simulink model "singlerobotlidarmap"  (R2021b)
settings: Solver=VariableStepAuto  StartTime=0.0  StopTime=10.0  RelTol=1e-3
InitFcn:
  | addpath("..");
  | initenv
libraries: mobileRoboticsLib x5, robotmobilelib x2
settings Model: Creator=yekin  LastModifiedBy=yekin

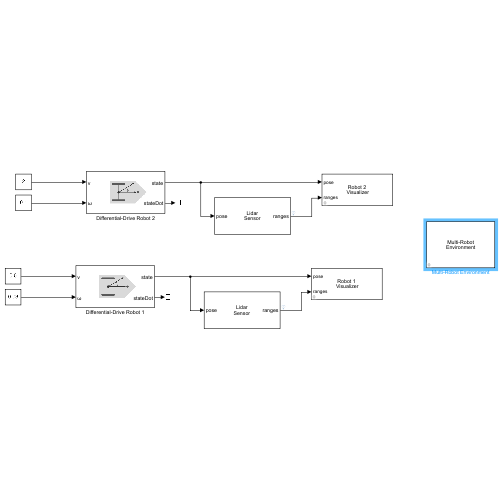
[thumbnail: Simulink's stored preview of the top-level diagram]
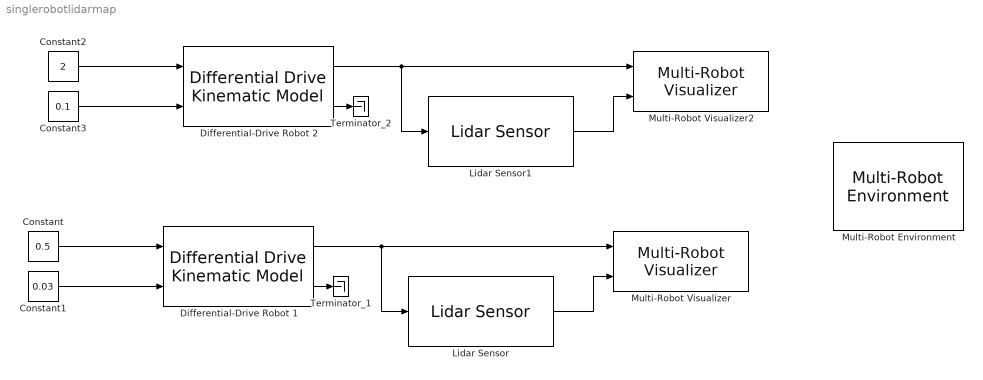
== system singlerobotlidarmap ==
  Constant : Constant  Value=0.5
  Constant1 : Constant  Value=0.03
  Constant2 : Constant  Value=2
  Constant3 : Constant  Value=0.1
  Differential-Drive Robot 1 : robotmobilelib/Differential Drive Kinematic Model  VehicleInputs=Vehicle Speed & Heading Angular Velocity  WheelRadius=0.3  WheelSpeedRange=[-pi pi]  TrackWidth=0.2  InitialState=[8, 19, 0.1]'  SimulateUsing=Interpreted execution
      settings: SourceProductBaseCode=RO
  Differential-Drive Robot 2 : robotmobilelib/Differential Drive Kinematic Model  VehicleInputs=Vehicle Speed & Heading Angular Velocity  WheelRadius=0.3  WheelSpeedRange=[-pi pi]  TrackWidth=0.2  InitialState=[15, 18, -0.3]'  SimulateUsing=Interpreted execution
      settings: SourceProductBaseCode=RO
  Lidar Sensor : mobileRoboticsLib/Environments/Lidar Sensor  mapName=map  sensorOffset=[ 0, 0 ]  scanAngles=[ -pi/4, 0, pi/4 ]  maxRange=20
      settings: SourceProductName=Mobile Robotics Simulation Toolbox
  Lidar Sensor1 : mobileRoboticsLib/Environments/Lidar Sensor  mapName=map  sensorOffset=[ 0, 0 ]  scanAngles=[ -pi/4, 0, pi/4 ]  maxRange=20
      settings: SourceProductName=Mobile Robotics Simulation Toolbox
  Multi-Robot Environment : mobileRoboticsLib/Environments/Multi-Robot Environment  numRobots=2  mapName=map  showWaypoints=off  showObjects=off  objectColors=[ 1, 0, 0; 0, 1, 0; 0, 0, 1 ]  objectMarkers='s'  showRobotIds=on  plotSensorLines=on
      settings: SourceProductName=Mobile Robotics Simulation Toolbox
  Multi-Robot Visualizer : mobileRoboticsLib/Environments/Multi-Robot Visualizer  idx=1  radius=0.3  robotColor=[0 0 1]  showTraj=on  hasLidar=on  sensorOffset=[0,0]  scanAngles=[-pi/4 0 pi/4]  maxNumScans=0  hasObjDetector=on  objDetectorOffset=[0,0]  objDetectorAngle=0  objDetectorFOV=pi/3  objDetectorMaxRange=2  hasRobotDetector=off  robotDetectorOffset=[0,0]  robotDetectorAngle=0  robotDetectorFOV=pi/3  robotDetectorMaxRange=5  robotDetectorNumDetections=0
      settings: SourceProductName=Mobile Robotics Simulation Toolbox
  Multi-Robot Visualizer2 : mobileRoboticsLib/Environments/Multi-Robot Visualizer  idx=2  radius=0.3  robotColor=[0 0 1]  showTraj=on  hasLidar=on  sensorOffset=[0,0]  scanAngles=[-pi/4 0 pi/4]  maxNumScans=0  hasObjDetector=off  objDetectorOffset=[0,0]  objDetectorAngle=0  objDetectorFOV=pi/3  objDetectorMaxRange=5  hasRobotDetector=on  robotDetectorOffset=[0,0]  robotDetectorAngle=0  robotDetectorFOV=pi/3  robotDetectorMaxRange=2  robotDetectorNumDetections=0
      settings: SourceProductName=Mobile Robotics Simulation Toolbox
  Terminator_1 : Terminator
  Terminator_2 : Terminator
  wires:
  Differential-Drive Robot 1/2 -> Terminator_1/1
  Constant1/1 -> Differential-Drive Robot 1/2
  Differential-Drive Robot 1/1 -> Multi-Robot Visualizer/1, Lidar Sensor/1
  Constant/1 -> Differential-Drive Robot 1/1
  Lidar Sensor/1 -> Multi-Robot Visualizer/2
  Constant2/1 -> Differential-Drive Robot 2/1
  Constant3/1 -> Differential-Drive Robot 2/2
  Lidar Sensor1/1 -> Multi-Robot Visualizer2/2
  Differential-Drive Robot 2/1 -> Multi-Robot Visualizer2/1, Lidar Sensor1/1
  Differential-Drive Robot 2/2 -> Terminator_2/1
